simulink model "computeFRI"  (Simulink 7.9)
settings: Solver=FixedStepDiscrete  StartTime=0.0  StopTime=20  FixedStep=0.010  RelTol=1e-3
InitFcn:
  | h=axes;
libraries: WBCLibrary x5
settings Model: Creator=jorhabib  LastModifiedBy=daniele
settings DataIOCC: SignalLoggingSaveFormat=Dataset
settings OptimizationCC: ExpressionDepthLimit=128
settings DebuggingCC: UnderspecifiedInitializationDetection=Simplified  StateNameClashWarn=none
settings CodeAppCC: CustomSymbolStrType=$N$R$M_T
settings GRTTargetCC: CodeReplacementLibrary=None  CPPClassGenCompliant=on

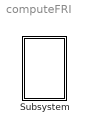
== system computeFRI ==
  Subsystem : Subsystem

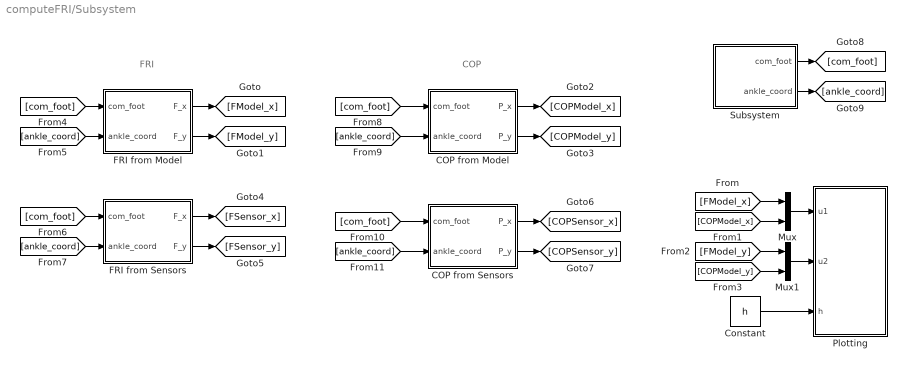
== system computeFRI/Subsystem ==
  note: COP
  note: FRI
  COP from Model : Subsystem  mask{robotName='iCubGenova01', localName='simulink', Ts=0.010}
      mask prompts: robotName "robot name"; localName "local name"
  COP from Sensors : Subsystem  mask{robotName='iCubGenova01', localName='simulink', Ts=0.010}
      mask prompts: robotName "robot name"; localName "local name"
  Constant : Constant  Value=h
  FRI from Model : Subsystem  mask{robotName='iCubGenova01', localName='simulink', Ts=0.010}
      mask prompts: robotName "robot name"; localName "local name"
  FRI from Sensors : Subsystem  mask{robotName='iCubGenova01', localName='simulink', Ts=0.010}
      mask prompts: robotName "robot name"; localName "local name"
  Mux : Mux  Inputs=2
  Mux1 : Mux  Inputs=2
  Plotting : MATLAB Function  TreatAsAtomicUnit=on
      settings: PermitHierarchicalResolution=ParametersOnly
  Subsystem : Subsystem  mask{robotName='iCubGenova01', localName='simulink', Ts=0.010}
      mask prompts: robotName "Robot name"; localName "Local name"
  wires:
  FRI from Model/1(F_x) -> [FModel_x]
  FRI from Model/2(F_y) -> [FModel_y]
  COP from Model/1(P_x) -> [COPModel_x]
  COP from Model/2(P_y) -> [COPModel_y]
  FRI from Sensors/1(F_x) -> [FSensor_x]
  FRI from Sensors/2(F_y) -> [FSensor_y]
  COP from Sensors/1(P_x) -> [COPSensor_x]
  COP from Sensors/2(P_y) -> [COPSensor_y]
  Subsystem/1(com_foot) -> [com_foot]
  Subsystem/2(ankle_coord) -> [ankle_coord]
  [com_foot] -> FRI from Model/1(com_foot)
  [ankle_coord] -> FRI from Model/2(ankle_coord)
  [com_foot] -> FRI from Sensors/1(com_foot)
  [ankle_coord] -> FRI from Sensors/2(ankle_coord)
  [ankle_coord] -> COP from Model/2(ankle_coord)
  [com_foot] -> COP from Model/1(com_foot)
  [ankle_coord] -> COP from Sensors/2(ankle_coord)
  [com_foot] -> COP from Sensors/1(com_foot)
  Constant/1 -> Plotting/3(h)
  [FModel_x] -> Mux/1
  [COPModel_x] -> Mux/2
  Mux/1 -> Plotting/1(u1)
  [FModel_y] -> Mux1/1
  [COPModel_y] -> Mux1/2
  Mux1/1 -> Plotting/2(u2)

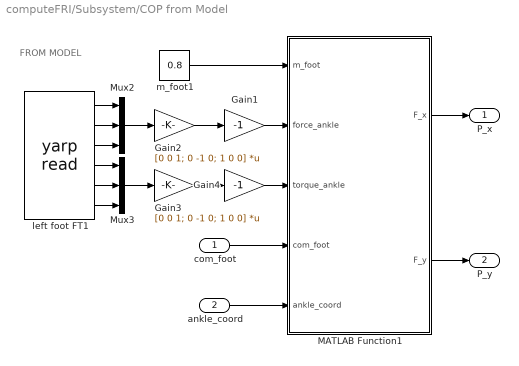
== system computeFRI/Subsystem/COP from Model ==
  note: FROM MODEL
  com_foot : Inport
  ankle_coord : Inport  Port=2
  Gain1 : Gain  Gain=-1  SampleTime=Ts
  Gain2 : Gain  Gain=[0 0 1; 0 -1 0; 1 0 0]  Multiplication=Matrix(K*u)  SampleTime=Ts
  Gain3 : Gain  Gain=[0 0 1; 0 -1 0; 1 0 0]  Multiplication=Matrix(K*u)  SampleTime=Ts
  Gain4 : Gain  Gain=-1  SampleTime=Ts
  MATLAB Function1 : MATLAB Function  TreatAsAtomicUnit=on
      settings: PermitHierarchicalResolution=ParametersOnly
  Mux2 : Mux  Inputs=3
  Mux3 : Mux  Inputs=3
  left foot FT1 : WBCLibrary/Utilities/yarp read  from='/wbdt/joint_foot_cartesian_wrench_from_model:o'  to='...'  num=6
  m_foot1 : Constant  Value=0.8  SampleTime=Ts
  P_x : Outport
  P_y : Outport  Port=2
  wires:
  MATLAB Function1/2(F_y) -> P_y/1
  Gain4/1 -> MATLAB Function1/3(torque_ankle)
  Gain1/1 -> MATLAB Function1/2(force_ankle)
  left foot FT1/4 -> Mux3/1
  MATLAB Function1/1(F_x) -> P_x/1
  left foot FT1/1 -> Mux2/1
  Mux3/1 -> Gain3/1
  Mux2/1 -> Gain2/1
  left foot FT1/3 -> Mux2/3
  left foot FT1/6 -> Mux3/3
  left foot FT1/5 -> Mux3/2
  Gain2/1 -> Gain1/1
  left foot FT1/2 -> Mux2/2
  Gain3/1 -> Gain4/1
  m_foot1/1 -> MATLAB Function1/1(m_foot)
  com_foot/1 -> MATLAB Function1/4(com_foot)
  ankle_coord/1 -> MATLAB Function1/5(ankle_coord)

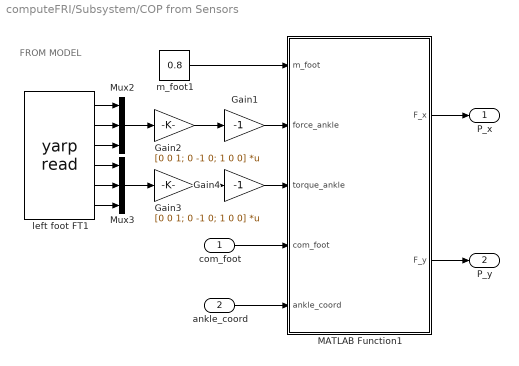
== system computeFRI/Subsystem/COP from Sensors ==
  note: FROM MODEL
  com_foot : Inport
  ankle_coord : Inport  Port=2
  Gain1 : Gain  Gain=-1  SampleTime=Ts
  Gain2 : Gain  Gain=[0 0 1; 0 -1 0; 1 0 0]  Multiplication=Matrix(K*u)  SampleTime=Ts
  Gain3 : Gain  Gain=[0 0 1; 0 -1 0; 1 0 0]  Multiplication=Matrix(K*u)  SampleTime=Ts
  Gain4 : Gain  Gain=-1  SampleTime=Ts
  MATLAB Function1 : MATLAB Function  TreatAsAtomicUnit=on
      settings: PermitHierarchicalResolution=ParametersOnly
  Mux2 : Mux  Inputs=3
  Mux3 : Mux  Inputs=3
  left foot FT1 : WBCLibrary/Utilities/yarp read  from='/wbdt/joint_foot_cartesian_wrench:o'  to='...'  num=6
  m_foot1 : Constant  Value=0.8  SampleTime=Ts
  P_x : Outport
  P_y : Outport  Port=2
  wires:
  m_foot1/1 -> MATLAB Function1/1(m_foot)
  Gain3/1 -> Gain4/1
  left foot FT1/2 -> Mux2/2
  Gain2/1 -> Gain1/1
  left foot FT1/5 -> Mux3/2
  left foot FT1/6 -> Mux3/3
  left foot FT1/3 -> Mux2/3
  Mux2/1 -> Gain2/1
  Mux3/1 -> Gain3/1
  left foot FT1/1 -> Mux2/1
  MATLAB Function1/1(F_x) -> P_x/1
  left foot FT1/4 -> Mux3/1
  Gain1/1 -> MATLAB Function1/2(force_ankle)
  Gain4/1 -> MATLAB Function1/3(torque_ankle)
  MATLAB Function1/2(F_y) -> P_y/1
  com_foot/1 -> MATLAB Function1/4(com_foot)
  ankle_coord/1 -> MATLAB Function1/5(ankle_coord)

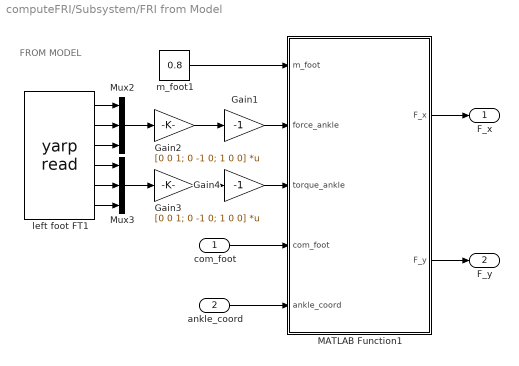
== system computeFRI/Subsystem/FRI from Model ==
  note: FROM MODEL
  com_foot : Inport
  ankle_coord : Inport  Port=2
  Gain1 : Gain  Gain=-1  SampleTime=Ts
  Gain2 : Gain  Gain=[0 0 1; 0 -1 0; 1 0 0]  Multiplication=Matrix(K*u)  SampleTime=Ts
  Gain3 : Gain  Gain=[0 0 1; 0 -1 0; 1 0 0]  Multiplication=Matrix(K*u)  SampleTime=Ts
  Gain4 : Gain  Gain=-1  SampleTime=Ts
  MATLAB Function1 : MATLAB Function  TreatAsAtomicUnit=on
      settings: PermitHierarchicalResolution=ParametersOnly
  Mux2 : Mux  Inputs=3
  Mux3 : Mux  Inputs=3
  left foot FT1 : WBCLibrary/Utilities/yarp read  from='/wbdt/joint_ankle_cartesian_wrench_from_model:o'  to='...'  num=6
  m_foot1 : Constant  Value=0.8  SampleTime=Ts
  F_x : Outport
  F_y : Outport  Port=2
  wires:
  m_foot1/1 -> MATLAB Function1/1(m_foot)
  Gain3/1 -> Gain4/1
  left foot FT1/2 -> Mux2/2
  Gain2/1 -> Gain1/1
  left foot FT1/5 -> Mux3/2
  left foot FT1/6 -> Mux3/3
  left foot FT1/3 -> Mux2/3
  Mux2/1 -> Gain2/1
  Mux3/1 -> Gain3/1
  left foot FT1/1 -> Mux2/1
  MATLAB Function1/1(F_x) -> F_x/1
  left foot FT1/4 -> Mux3/1
  Gain1/1 -> MATLAB Function1/2(force_ankle)
  Gain4/1 -> MATLAB Function1/3(torque_ankle)
  MATLAB Function1/2(F_y) -> F_y/1
  com_foot/1 -> MATLAB Function1/4(com_foot)
  ankle_coord/1 -> MATLAB Function1/5(ankle_coord)

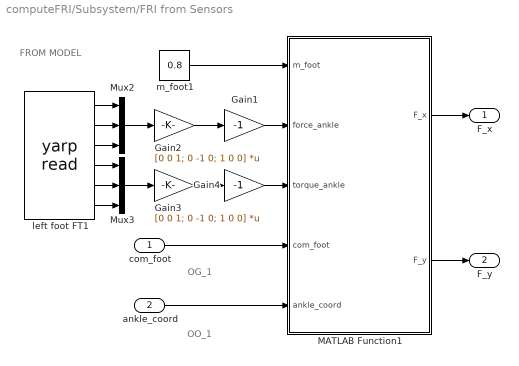
== system computeFRI/Subsystem/FRI from Sensors ==
  note: OO_1
  note: OG_1
  note: FROM MODEL
  com_foot : Inport
  ankle_coord : Inport  Port=2
  Gain1 : Gain  Gain=-1  SampleTime=Ts
  Gain2 : Gain  Gain=[0 0 1; 0 -1 0; 1 0 0]  Multiplication=Matrix(K*u)  SampleTime=Ts
  Gain3 : Gain  Gain=[0 0 1; 0 -1 0; 1 0 0]  Multiplication=Matrix(K*u)  SampleTime=Ts
  Gain4 : Gain  Gain=-1  SampleTime=Ts
  MATLAB Function1 : MATLAB Function  TreatAsAtomicUnit=on
      settings: PermitHierarchicalResolution=ParametersOnly
  Mux2 : Mux  Inputs=3
  Mux3 : Mux  Inputs=3
  left foot FT1 : WBCLibrary/Utilities/yarp read  from='/wbdt/joint_ankle_cartesian_wrench:o'  to='...'  num=6
  m_foot1 : Constant  Value=0.8  SampleTime=Ts
  F_x : Outport
  F_y : Outport  Port=2
  wires:
  MATLAB Function1/2(F_y) -> F_y/1
  Gain4/1 -> MATLAB Function1/3(torque_ankle)
  Gain1/1 -> MATLAB Function1/2(force_ankle)
  left foot FT1/4 -> Mux3/1
  MATLAB Function1/1(F_x) -> F_x/1
  left foot FT1/1 -> Mux2/1
  Mux3/1 -> Gain3/1
  Mux2/1 -> Gain2/1
  left foot FT1/3 -> Mux2/3
  left foot FT1/6 -> Mux3/3
  left foot FT1/5 -> Mux3/2
  Gain2/1 -> Gain1/1
  left foot FT1/2 -> Mux2/2
  Gain3/1 -> Gain4/1
  m_foot1/1 -> MATLAB Function1/1(m_foot)
  com_foot/1 -> MATLAB Function1/4(com_foot)
  ankle_coord/1 -> MATLAB Function1/5(ankle_coord)

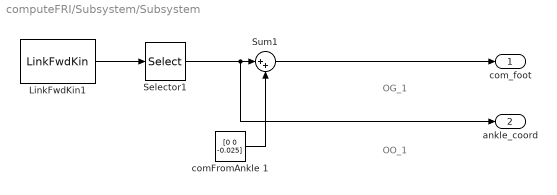
== system computeFRI/Subsystem/Subsystem ==
  note: OG_1
  note: OO_1
  LinkFwdKin1 : WBCLibrary/wholeBodyModel/Forward Kinematics/LinkFwdKin  robotname=robotName  localname=localName  link=l_ankle_1
  Selector1 : Selector  InputPortWidth=7  IndexOptions=Index vector (dialog)  Indices=[1:3]  OutputSizes=1
  Sum1 : Sum  Inputs=|++  SampleTime=Ts
  comFromAnkle 1 : Constant  Value=[0 0 -0.025]  SampleTime=Ts
  com_foot : Outport
  ankle_coord : Outport  Port=2
  wires:
  Selector1/1 -> ankle_coord/1, Sum1/1
  comFromAnkle 1/1 -> Sum1/2
  Sum1/1 -> com_foot/1
  LinkFwdKin1/1 -> Selector1/1

== matlab function Subsystem/FRI from Model/MATLAB Function1 ==
  data: F_x output double; m_foot input double; force_ankle input double; torque_ankle input double; com_foot input double; ankle_coord input double; F_y output double
function [F_x, F_y] = SOF(m_foot, force_ankle, torque_ankle, com_foot, ankle_coord)
%#codegen

grav = [0 0 -9.8]';
g_z = abs(grav(3));
% S_OF = (1/norm(m_foot*grav - force_ankle)^2) * (Sf(com_foot)*m_foot*grav - Sf(ankle_coord)*force_ankle - torque_ankle)*(m_foot*grav - force_ankle)'
% 
% y = S_OF;


F_x = (-torque_ankle(2) - ankle_coord(3)*force_ankle(1) + ankle_coord(1)*force_ankle(3) + m_foot*g_z*com_foot(1)) / (m_foot*g_z + force_ankle(3));
F_y = ( torque_ankle(1) - ankle_coord(3)*force_ankle(2) + ankle_coord(2)*force_ankle(3) + m_foot*g_z*com_foot(2)) / (m_foot*g_z + force_ankle(3));

== matlab function Subsystem/FRI from Sensors/MATLAB Function1 ==
  data: F_x output double; m_foot input double; force_ankle input double; torque_ankle input double; com_foot input double; ankle_coord input double; F_y output double
function [F_x, F_y] = SOF(m_foot, force_ankle, torque_ankle, com_foot, ankle_coord)
%#codegen

grav = [0 0 -9.8]';
g_z = abs(grav(3));
% S_OF = (1/norm(m_foot*grav - force_ankle)^2) * (Sf(com_foot)*m_foot*grav - Sf(ankle_coord)*force_ankle - torque_ankle)*(m_foot*grav - force_ankle)'
% 
% y = S_OF;


F_x = (-torque_ankle(2) - ankle_coord(3)*force_ankle(1) + ankle_coord(1)*force_ankle(3) + m_foot*g_z*com_foot(1)) / (m_foot*g_z + force_ankle(3));
F_y = ( torque_ankle(1) - ankle_coord(3)*force_ankle(2) + ankle_coord(2)*force_ankle(3) + m_foot*g_z*com_foot(2)) / (m_foot*g_z + force_ankle(3));

== matlab function Subsystem/COP from Model/MATLAB Function1 ==
  data: F_x output double; m_foot input double; force_ankle input double; torque_ankle input double; com_foot input double; ankle_coord input double; F_y output double
function [F_x, F_y] = SOF(m_foot, force_ankle, torque_ankle, com_foot, ankle_coord)
%#codegen

grav = [0 0 -9.8]';
g_z = abs(grav(3));
% S_OF = (1/norm(m_foot*grav - force_ankle)^2) * (Sf(com_foot)*m_foot*grav - Sf(ankle_coord)*force_ankle - torque_ankle)*(m_foot*grav - force_ankle)'
% 
% y = S_OF;


F_x = (-torque_ankle(2) - ankle_coord(3)*force_ankle(1) + ankle_coord(1)*force_ankle(3) + m_foot*g_z*com_foot(1)) / (m_foot*g_z + force_ankle(3));
F_y = ( torque_ankle(1) - ankle_coord(3)*force_ankle(2) + ankle_coord(2)*force_ankle(3) + m_foot*g_z*com_foot(2)) / (m_foot*g_z + force_ankle(3));

== matlab function Subsystem/COP from Sensors/MATLAB Function1 ==
  data: F_x output double; m_foot input double; force_ankle input double; torque_ankle input double; com_foot input double; ankle_coord input double; F_y output double
function [F_x, F_y] = SOF(m_foot, force_ankle, torque_ankle, com_foot, ankle_coord)
%#codegen

grav = [0 0 -9.8]';
g_z = abs(grav(3));
% S_OF = (1/norm(m_foot*grav - force_ankle)^2) * (Sf(com_foot)*m_foot*grav - Sf(ankle_coord)*force_ankle - torque_ankle)*(m_foot*grav - force_ankle)'
% 
% y = S_OF;


F_x = (-torque_ankle(2) - ankle_coord(3)*force_ankle(1) + ankle_coord(1)*force_ankle(3) + m_foot*g_z*com_foot(1)) / (m_foot*g_z + force_ankle(3));
F_y = ( torque_ankle(1) - ankle_coord(3)*force_ankle(2) + ankle_coord(2)*force_ankle(3) + m_foot*g_z*com_foot(2)) / (m_foot*g_z + force_ankle(3));

== matlab function Subsystem/Plotting ==
  data: u1 input double; u2 input double; h input double
function fcn(u1, u2, h)
%#codegen

% plot(h,u1(1),u2(1),'b.');
% hold on;
% plot(h,u1(2),u2(2),'r.');
% axis equal;

line([u1(1),u1(1)],[u2(1),u2(1)],'LineStyle','none','Marker','o','MarkerEdge','b','MarkerSize',3);
hold on;
line([u1(2),u1(2)],[u2(2),u2(2)],'LineStyle','none','Marker','o','MarkerEdge','r','MarkerSize',3);
axis equal;
